simulink library "SMXL"  (Simulink 2.3)
libraries: smxl x55, SMXL x9, simulink3 x4
(part 2 of 2)

== system SMXL/Rotation Matrices/Euler/Earth2Kine/Tfb ==
  mu : Inport  Port=1  PortWidth=-1  SampleTime=-1  DataType=auto
      settings: SignalType=auto
  Constant : Constant  Value=0
  Constant3 : Constant  Value=1
  Gain : Gain  Gain=-1  SaturateOnIntegerOverflow=on
  Mux : Mux  Inputs=9
  Trigonometric Function1 : Trigonometry  Operator=cos  OutputSignalType=auto
  Trigonometric Function2 : Trigonometry  Operator=sin  OutputSignalType=auto
  Tfb : Outport  Port=1
  wires:
  Trigonometric Function1/1 -> Mux/9, Mux/5
  Gain/1 -> Mux/8
  Trigonometric Function2/1 -> Gain/1, Mux/6
  mu/1 -> Trigonometric Function2/1, Trigonometric Function1/1
  Constant/1 -> Mux/7, Mux/4, Mux/3, Mux/2
  Constant3/1 -> Mux/1
  Mux/1 -> Tfb/1

== system SMXL/Rotation Matrices/Euler/Earth2Kine/Toc ==
  chi : Inport  Port=1  PortWidth=-1  SampleTime=-1  DataType=auto
      settings: SignalType=auto
  Constant : Constant  Value=0
  Constant2 : Constant  Value=1
  Gain : Gain  Gain=-1  SaturateOnIntegerOverflow=on
  Mux : Mux  Inputs=9
  Trigonometric Function1 : Trigonometry  Operator=cos  OutputSignalType=auto
  Trigonometric Function2 : Trigonometry  Operator=sin  OutputSignalType=auto
  Toc : Outport  Port=1
  wires:
  Mux/1 -> Toc/1
  Constant/1 -> Mux/6, Mux/8, Mux/7, Mux/3
  Constant2/1 -> Mux/9
  Gain/1 -> Mux/4
  Trigonometric Function2/1 -> Mux/2, Gain/1
  Trigonometric Function1/1 -> Mux/5, Mux/1
  chi/1 -> Trigonometric Function2/1, Trigonometric Function1/1

== system SMXL/Rotation Matrices/Euler/Kine2Earth/Tcf ==
  gamma : Inport  Port=1  PortWidth=-1  SampleTime=-1  DataType=auto
      settings: SignalType=auto
  Constant : Constant  Value=0
  Constant2 : Constant  Value=1
  Gain : Gain  Gain=-1  SaturateOnIntegerOverflow=on
  Mux : Mux  Inputs=9
  Trigonometric Function1 : Trigonometry  Operator=cos  OutputSignalType=auto
  Trigonometric Function2 : Trigonometry  Operator=sin  OutputSignalType=auto
  Tcf : Outport  Port=1
  wires:
  Trigonometric Function1/1 -> Mux/9, Mux/1
  Trigonometric Function2/1 -> Mux/7, Gain/1
  Constant2/1 -> Mux/5
  Constant/1 -> Mux/8, Mux/6, Mux/4, Mux/2
  Gain/1 -> Mux/3
  gamma/1 -> Trigonometric Function1/1, Trigonometric Function2/1
  Mux/1 -> Tcf/1

== system SMXL/Rotation Matrices/Euler/Kine2Earth/Tfb ==
  mu : Inport  Port=1  PortWidth=-1  SampleTime=-1  DataType=auto
      settings: SignalType=auto
  Constant : Constant  Value=0
  Constant3 : Constant  Value=1
  Gain : Gain  Gain=-1  SaturateOnIntegerOverflow=on
  Mux : Mux  Inputs=9
  Trigonometric Function1 : Trigonometry  Operator=cos  OutputSignalType=auto
  Trigonometric Function2 : Trigonometry  Operator=sin  OutputSignalType=auto
  Tfb : Outport  Port=1
  wires:
  Trigonometric Function1/1 -> Mux/9, Mux/5
  Gain/1 -> Mux/8
  Trigonometric Function2/1 -> Gain/1, Mux/6
  mu/1 -> Trigonometric Function2/1, Trigonometric Function1/1
  Constant/1 -> Mux/7, Mux/4, Mux/3, Mux/2
  Constant3/1 -> Mux/1
  Mux/1 -> Tfb/1

== system SMXL/Rotation Matrices/Euler/Kine2Earth/Toc ==
  chi : Inport  Port=1  PortWidth=-1  SampleTime=-1  DataType=auto
      settings: SignalType=auto
  Constant : Constant  Value=0
  Constant2 : Constant  Value=1
  Gain : Gain  Gain=-1  SaturateOnIntegerOverflow=on
  Mux : Mux  Inputs=9
  Trigonometric Function1 : Trigonometry  Operator=cos  OutputSignalType=auto
  Trigonometric Function2 : Trigonometry  Operator=sin  OutputSignalType=auto
  Toc : Outport  Port=1
  wires:
  Mux/1 -> Toc/1
  Constant/1 -> Mux/6, Mux/8, Mux/7, Mux/3
  Constant2/1 -> Mux/9
  Gain/1 -> Mux/4
  Trigonometric Function2/1 -> Mux/2, Gain/1
  Trigonometric Function1/1 -> Mux/5, Mux/1
  chi/1 -> Trigonometric Function2/1, Trigonometric Function1/1

== system SMXL/Rotation Matrices/Euler/Wind2Body/Tcf ==
  alpha : Inport  Port=1  PortWidth=-1  SampleTime=-1  DataType=auto
      settings: SignalType=auto
  Constant : Constant  Value=0
  Constant2 : Constant  Value=1
  Gain : Gain  Gain=-1  SaturateOnIntegerOverflow=on
  Mux : Mux  Inputs=9
  Trigonometric Function1 : Trigonometry  Operator=cos  OutputSignalType=auto
  Trigonometric Function2 : Trigonometry  Operator=sin  OutputSignalType=auto
  Tcf : Outport  Port=1
  wires:
  Trigonometric Function1/1 -> Mux/9, Mux/1
  Trigonometric Function2/1 -> Mux/7, Gain/1
  Constant2/1 -> Mux/5
  Constant/1 -> Mux/8, Mux/6, Mux/4, Mux/2
  Gain/1 -> Mux/3
  alpha/1 -> Trigonometric Function1/1, Trigonometric Function2/1
  Mux/1 -> Tcf/1

== system SMXL/Rotation Matrices/Euler/Wind2Body/Toc ==
  beta : Inport  Port=1  PortWidth=-1  SampleTime=-1  DataType=auto
      settings: SignalType=auto
  Constant : Constant  Value=0
  Constant2 : Constant  Value=1
  Gain : Gain  Gain=-1  SaturateOnIntegerOverflow=on
  Mux : Mux  Inputs=9
  Trigonometric Function1 : Trigonometry  Operator=cos  OutputSignalType=auto
  Trigonometric Function2 : Trigonometry  Operator=sin  OutputSignalType=auto
  Toc : Outport  Port=1
  wires:
  Mux/1 -> Toc/1
  Constant/1 -> Mux/6, Mux/8, Mux/7, Mux/3
  Constant2/1 -> Mux/9
  Gain/1 -> Mux/4
  Trigonometric Function2/1 -> Mux/2, Gain/1
  Trigonometric Function1/1 -> Mux/5, Mux/1
  beta/1 -> Trigonometric Function2/1, Trigonometric Function1/1

== system SMXL/Rotation Matrices/Quaternions/Body2Earth/Subsystem ==
  In1 : Inport  Port=1  PortWidth=-1  SampleTime=-1  DataType=auto
      settings: SignalType=auto
  State Space : StateSpace  A=[]  B=[]  C=[]  D=[0 0 0;0 0 1;0 -1 0;0 0 -1;0 0 0;1 0 0;0 1 0;-1 0 0;0 0 0]  X0=0
  Out1 : Outport  Port=1
  wires:
  In1/1 -> State Space/1
  State Space/1 -> Out1/1

== system SMXL/Rotation Matrices/Quaternions/Earth2Body/Subsystem ==
  In1 : Inport  Port=1  PortWidth=-1  SampleTime=-1  DataType=auto
      settings: SignalType=auto
  State Space : StateSpace  A=[]  B=[]  C=[]  D=[0 0 0;0 0 1;0 -1 0;0 0 -1;0 0 0;1 0 0;0 1 0;-1 0 0;0 0 0]  X0=0
  Out1 : Outport  Port=1
  wires:
  State Space/1 -> Out1/1
  In1/1 -> State Space/1

== system SMXL/Rotation Matrices/Quaternions/endot2pqr/Subsystem ==
  In1 : Inport  Port=1  PortWidth=-1  SampleTime=-1  DataType=auto
      settings: SignalType=auto
  State Space : StateSpace  A=[]  B=[]  C=[]  D=[0 0 0;0 0 1;0 -1 0;0 0 -1;0 0 0;1 0 0;0 1 0;-1 0 0;0 0 0]  X0=0
  Out1 : Outport  Port=1
  wires:
  State Space/1 -> Out1/1
  In1/1 -> State Space/1

== system SMXL/Rotation Matrices/Quaternions/endot2pqr/Subsystem1 ==
  In1 : Inport  Port=1  PortWidth=-1  SampleTime=-1  DataType=auto
      settings: SignalType=auto
  State Space : StateSpace  A=[]  B=[]  C=[]  D=[1 0 0 0 1 0 0 0 1]'  X0=0
  Out1 : Outport  Port=1
  wires:
  In1/1 -> State Space/1
  State Space/1 -> Out1/1

== system SMXL/Rotation Matrices/Quaternions/pqr2endot/Subsystem ==
  In1 : Inport  Port=1  PortWidth=-1  SampleTime=-1  DataType=auto
      settings: SignalType=auto
  State Space : StateSpace  A=[]  B=[]  C=[]  D=[0 0 0;0 0 1;0 -1 0;0 0 -1;0 0 0;1 0 0;0 1 0;-1 0 0;0 0 0]  X0=0
  Out1 : Outport  Port=1
  wires:
  State Space/1 -> Out1/1
  In1/1 -> State Space/1

== system SMXL/Rotation Matrices/Quaternions/pqr2endot/Subsystem1 ==
  In1 : Inport  Port=1  PortWidth=-1  SampleTime=-1  DataType=auto
      settings: SignalType=auto
  State Space : StateSpace  A=[]  B=[]  C=[]  D=[1 0 0 0 1 0 0 0 1]'  X0=0
  Out1 : Outport  Port=1
  wires:
  In1/1 -> State Space/1
  State Space/1 -> Out1/1
